simulink model "Problem1"  (R2020b)
settings: Solver=VariableStepAuto  StartTime=0.0  StopTime=100  RelTol=1e-3
values from neighbouring files (symbols this model uses):
  b = 50    [Parameters.m]
  K1 = 50    [Parameters.m]
  k12 = 25    [Parameters.m]
  M1 = 100    [Parameters.m]
  M2 = 50    [Parameters.m]
settings Model: Creator=adity  LastModifiedBy=adity

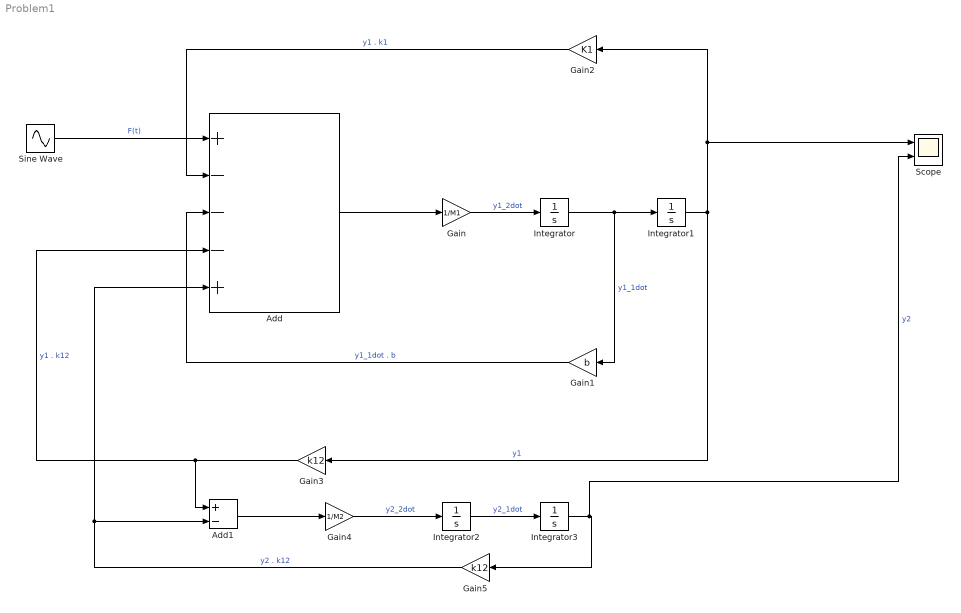
== system Problem1 ==
  Add : Sum  Inputs=+---+
  Add1 : Sum  Inputs=+-
  Gain : Gain  Gain=1/M1
  Gain1 : Gain  Gain=b
  Gain2 : Gain  Gain=K1
  Gain3 : Gain  Gain=k12
  Gain4 : Gain  Gain=1/M2
  Gain5 : Gain  Gain=k12
  Integrator{,1..3} (4 alike) : Integrator
  Scope : Scope  NumInputPorts=2
  Sine Wave : Sin  Amplitude=2  Frequency=10  SampleTime=0
  wires:
  Integrator2/1 -> Integrator3/1  "y2_1dot"
  Add/1 -> Gain/1
  Gain5/1 -> Add1/2, Add/5  "y2 . k12"
  Integrator3/1 -> Scope/2, Gain5/1  "y2"
  Gain2/1 -> Add/2  "y1 . k1"
  Sine Wave/1 -> Add/1  "F(t)"
  Gain3/1 -> Add/4, Add1/1  "y1 . k12"
  Integrator1/1 -> Gain3/1, Scope/1, Gain2/1  "y1"
  Gain/1 -> Integrator/1  "y1_2dot"
  Integrator/1 -> Gain1/1, Integrator1/1  "y1_1dot"
  Gain4/1 -> Integrator2/1  "y2_2dot"
  Add1/1 -> Gain4/1
  Gain1/1 -> Add/3  "y1_1dot . b"
